simulink model "LM_TOS_0115"  (R2018b)
settings: Solver=FixedStepDiscrete  StartTime=0.0  StopTime=inf  FixedStep=0.005  RelTol=1e-3
PostLoadFcn:
  | if any(exist('dsrtsu_mdlpostloadfcn', 'file') ~= 0), dsrtsu_mdlpostloadfcn('Execute', bdroot); end
(part 1 of 4)
settings Model: DSRTSU_INTERNAL_RTI_VER=540  DSRTSU_INTERNAL_RTI_TYPE=rti1401  RTICANMMDATA=struct('GeneralSetupData',struct('modelroot','D:\00_Work\00_ZOP\00_ZOP_Demo_sim\LaneModel_20210114_CYX_Fix_HWA_TAR_OBJ','generalsettings',struct('filesettings',struct('destfolder',struct('Name','RTICANMM_FILES','Check',1),'buildfolder',struct('Name','.','Check',1),'AbsDestfolder',struct('Name','D:\00_Work\00_ZOP\00_ZOP_Demo_sim\LaneModel_20210114_CYX_Fix_HWA_TAR_OBJ\RTICANMM_FILES'),'AbsBuildfolder',struct('Name','D:\00_Work\00_ZOP\00_ZOP_Demo_sim\LaneModel_20210114_CYX_Fix_HWA_TAR_OBJ'))),'options',struct('addpaths',1,'rmpaths',1,'addtrcexclusion',logical(1),'cannavigator',struct('checkmonitoring',0),'show_usrtrc',0,'use_usrtrc',0),'advanced',struct('options',ones(1,100)),'MPSetup',{{}},'RTI',struct('Type','RTI1401','Ver','7.12','Date','02-May-2019'),'modelname','LM_TOS','block','LM_TOS'))  DSRTSU_INTERNAL_RTIFPGA=130  Creator=only  LastModifiedBy=only
settings OptimizationCC: BlockReduction=off  ConditionallyExecuteInputs=off  DefaultUnderspecifiedDataType=single  BufferReuse=off  EnhancedBackFolding=on  ExpressionFolding=off  PassReuseOutputArgsThreshold=0  LocalBlockOutputs=off  OptimizeBlockOrder=speed  DifferentSizesBufferReuse=on
settings DebuggingCC: ParameterTunabilityLossMsg=error
settings HardwareCC: ProdBitPerPointer=32  ProdBitPerSizeT=32  ProdBitPerPtrDiffT=32  ProdLargestAtomicInteger=Integer  ProdEndianess=BigEndian  ProdWordSize=32  ProdHWDeviceType=Custom Processor->Custom  TargetIntDivRoundTo=Zero  TargetEndianess=BigEndian  TargetHWDeviceType=Custom Processor->Custom
settings ModelReferenceCC: ModelReferenceNumInstancesAllowed=Single
settings SFSimCC: MATLABDynamicMemAlloc=off
settings RTWCC: SystemTargetFile=rti1401.tlc  MakeCommand=make_rti  TemplateMakefile=rti1401.tmf  Description=dSPACE DS1401 Hardware Platform  GenerateReport=on  LaunchReport=on
settings CodeAppCC: OperatorAnnotations=on
settings STFCustomTargetCC: ParMdlRefBuildCompliant=on  SystemTargetFile=rti1401.tlc
settings GRTTargetCC: TargetLangStandard=C89/C90 (ANSI)  CompOptLevelCompliant=off  ConcurrentExecutionCompliant=off  CombineOutputUpdateFcns=off  MatFileLogging=off  CPPClassGenCompliant=off  UseToolchainInfoCompliant=off

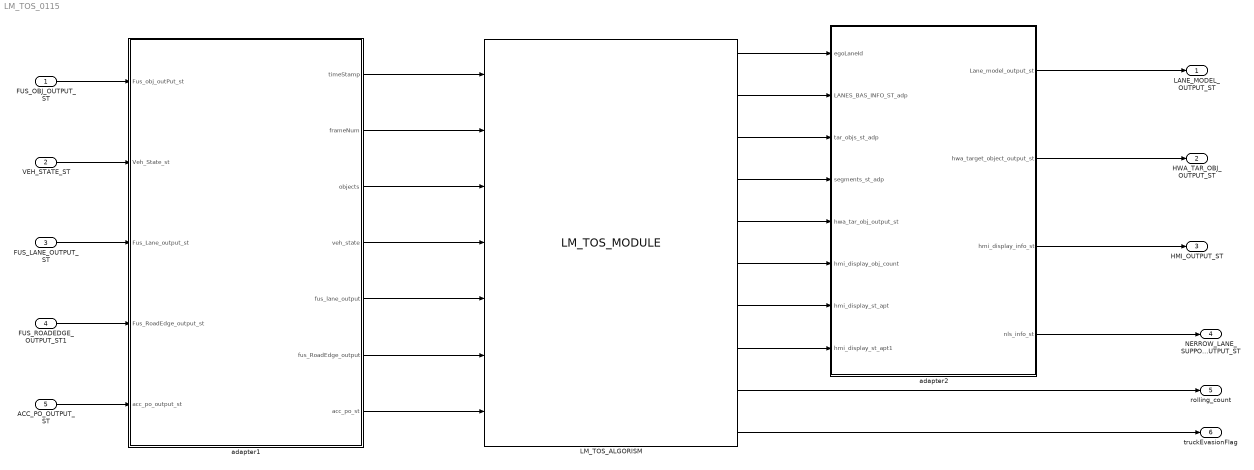
== system LM_TOS_0115 ==
  FUS_OBJ_OUTPUT_ST : Inport  OutDataTypeStr=Bus: FUS_OBJ_OUTPUT_ST
  VEH_STATE_ST : Inport  Port=2  OutDataTypeStr=Bus: VSI_VEHSTATE_ST
  FUS_LANE_OUTPUT_ST : Inport  Port=3  OutDataTypeStr=Bus: FUS_LANE_OUTPUT_ST
  FUS_ROADEDGE_OUTPUT_ST1 : Inport  Port=4  OutDataTypeStr=Bus: FUS_ROAD_EDGE_OUTPUT_ST
  ACC_PO_OUTPUT_ST : Inport  Port=5  OutDataTypeStr=Bus: ATS_PO_ST
  LM_TOS_ALGORISM : S-Function  InitFcn=try, set_param(gcb,'FunctionName','LM_TOS_MODULE'), end  FunctionName=LM_TOS_MODULE  SFunctionModules=LM_TOS_MODULE_wrapper Adapters LMBase LMMathLib LMPp LMTOSRunAlgo LMF TOSBase TOSHWA TOSPp VSL TOSNRA TOSTruckEvasion HMI CoordinationTransformation Parameters VehicleMovement DrivingManeuver LMCommonDefines  SFunctionDeploymentMode=off  EnableBusSupport=off  mask(S-Function Builder){}
      mask help: Simulink:masks:SFunctionBuilder_MD
      mask init:
      | val = [[.9  0.75 0.75 1 1 .9 .9 1]',[1 1 0.75 0.75 .9 .9 1 .9]'];try , sys = get_param(gcb,'SfunBuilderFcnName');if isempty(sys), sys = get_param(gcb,'FunctionName'); end,catch, sys = get_param(gcb,'FunctionName'); end
      settings: CopyFcn=set_param(gcbh,'LinkStatus','none')  PreSaveFcn=try, set_param(gcb,'FunctionName','LM_TOS_MODULE'), end  OpenFcn=sfunctionwizard(gcbh)
      mask Display: plot(val(:,1),val(:,2)),disp(sys), port_label('input',1,'timeStamp_In'), port_label('input',2,'frameNum_In'), port_label('input',3,'objects_In'), port_label('input',4,'vehState_In'), port_label('input',5,'fus_Lane_In'), port_label('input',6,'fus_roadEdge_In'), port_label('input',7,'acc_to_In'), port_label('output',1,'egoLaneId_output'), port_label('output',2,'lanes_bas_info_st_output'), port_label('output',3,'tar_obj_st_output'), port_label('output',4,'segments_st_output'), port_label('output',5,'hwa_tar_obj_st_output'), port_label('output',6,'hmi_obj_count_output'), port_label('output',7,'hmi_info_st_output'), port_label('output',8,'nls_info_st_output'), port_label('output',9,'rolling_count_output'), port_label('output',10,'te_Flag_output')
  adapter1 : Subsystem
  adapter2 : Subsystem
  LANE_MODEL_OUTPUT_ST : Outport  OutDataTypeStr=Bus: LANEMODEL_OUTPUT_ST
  HWA_TAR_OBJ_OUTPUT_ST : Outport  Port=2  OutDataTypeStr=Bus: HWA_TARGETOBJECT_OUTPUT_ST
  HMI_OUTPUT_ST : Outport  Port=3  OutDataTypeStr=Bus: HMI_OUTPUT_ST
  NERROW_LANE_SUPPORT_OUTPUT_ST : Outport  Port=4  OutDataTypeStr=Bus: NARROW_LANE_SUPPORT_OUTPUT_ST
  rolling_count : Outport  Port=5  OutDataTypeStr=uint16
  truckEvasionFlag : Outport  Port=6  OutDataTypeStr=uint8
  wires:
  LM_TOS_ALGORISM/4 -> adapter2/4(segments_st_adp)
  adapter2/2(hwa_target_object_output_st) -> HWA_TAR_OBJ_OUTPUT_ST/1
  adapter1/5(fus_lane_output) -> LM_TOS_ALGORISM/5
  adapter1/2(frameNum) -> LM_TOS_ALGORISM/2
  adapter1/3(objects) -> LM_TOS_ALGORISM/3
  FUS_OBJ_OUTPUT_ST/1 -> adapter1/1(Fus_obj_outPut_st)
  adapter1/1(timeStamp) -> LM_TOS_ALGORISM/1
  adapter1/4(veh_state) -> LM_TOS_ALGORISM/4
  adapter2/1(Lane_model_output_st) -> LANE_MODEL_OUTPUT_ST/1
  LM_TOS_ALGORISM/2 -> adapter2/2(LANES_BAS_INFO_ST_adp)
  FUS_LANE_OUTPUT_ST/1 -> adapter1/3(Fus_Lane_output_st)
  adapter1/7(acc_po_st) -> LM_TOS_ALGORISM/7
  adapter2/4(nls_info_st) -> NERROW_LANE_SUPPORT_OUTPUT_ST/1
  LM_TOS_ALGORISM/10 -> truckEvasionFlag/1
  LM_TOS_ALGORISM/9 -> rolling_count/1
  LM_TOS_ALGORISM/7 -> adapter2/7(hmi_display_st_apt)
  LM_TOS_ALGORISM/6 -> adapter2/6(hmi_display_obj_count)
  LM_TOS_ALGORISM/1 -> adapter2/1(egoLaneId)
  ACC_PO_OUTPUT_ST/1 -> adapter1/5(acc_po_output_st)
  LM_TOS_ALGORISM/3 -> adapter2/3(tar_objs_st_adp)
  adapter2/3(hmi_display_info_st) -> HMI_OUTPUT_ST/1
  LM_TOS_ALGORISM/8 -> adapter2/8(hmi_display_st_apt1)
  adapter1/6(fus_RoadEdge_output) -> LM_TOS_ALGORISM/6
  VEH_STATE_ST/1 -> adapter1/2(Veh_State_st)
  FUS_ROADEDGE_OUTPUT_ST1/1 -> adapter1/4(Fus_RoadEdge_output_st)
  LM_TOS_ALGORISM/5 -> adapter2/5(hwa_tar_obj_output_st)

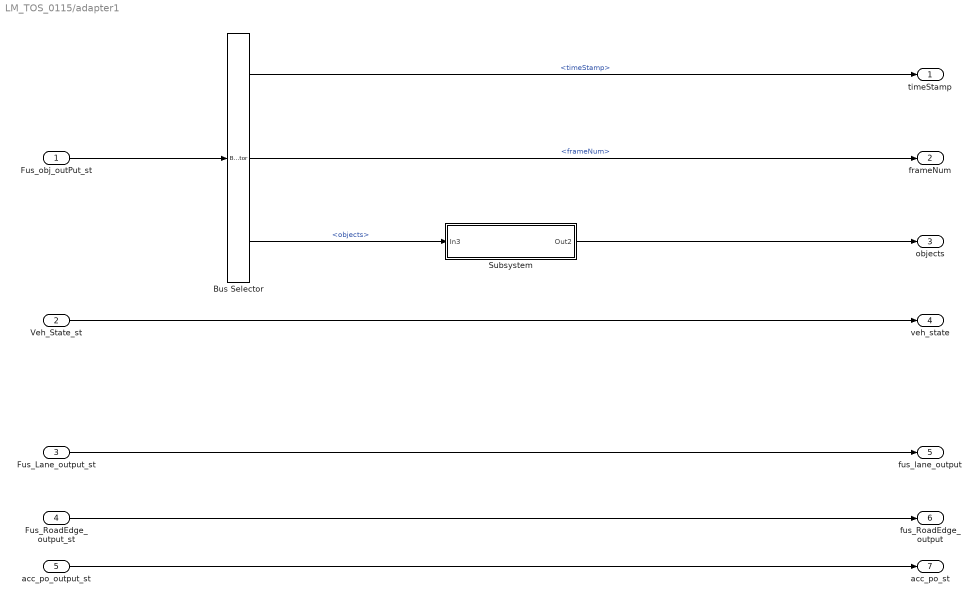
== system LM_TOS_0115/adapter1 ==
  Fus_obj_outPut_st : Inport  OutDataTypeStr=Bus: FUS_OBJ_OUTPUT_ST
  Veh_State_st : Inport  Port=2  OutDataTypeStr=Bus: VSI_VEHSTATE_ST
  Fus_Lane_output_st : Inport  Port=3  OutDataTypeStr=Bus: FUS_LANE_OUTPUT_ST
  Fus_RoadEdge_output_st : Inport  Port=4  OutDataTypeStr=Bus: FUS_ROAD_EDGE_OUTPUT_ST
  acc_po_output_st : Inport  Port=5  OutDataTypeStr=Bus: ATS_PO_ST
  Bus Selector : BusSelector  OutputSignals=timeStamp,frameNum,objects
  Subsystem : Subsystem
  timeStamp : Outport
  frameNum : Outport  Port=2
  objects : Outport  Port=3
  veh_state : Outport  Port=4
  fus_lane_output : Outport  Port=5
  fus_RoadEdge_output : Outport  Port=6  OutDataTypeStr=Bus: FUS_ROAD_EDGE_OUTPUT_ST
  acc_po_st : Outport  Port=7  OutDataTypeStr=Bus: ATS_PO_ST
  wires:
  Fus_obj_outPut_st/1 -> Bus Selector/1
  Bus Selector/3 -> Subsystem/1(In3)  "<objects>"
  Bus Selector/1 -> timeStamp/1  "<timeStamp>"
  Bus Selector/2 -> frameNum/1  "<frameNum>"
  Subsystem/1(Out2) -> objects/1
  Veh_State_st/1 -> veh_state/1
  Fus_Lane_output_st/1 -> fus_lane_output/1
  Fus_RoadEdge_output_st/1 -> fus_RoadEdge_output/1
  acc_po_output_st/1 -> acc_po_st/1

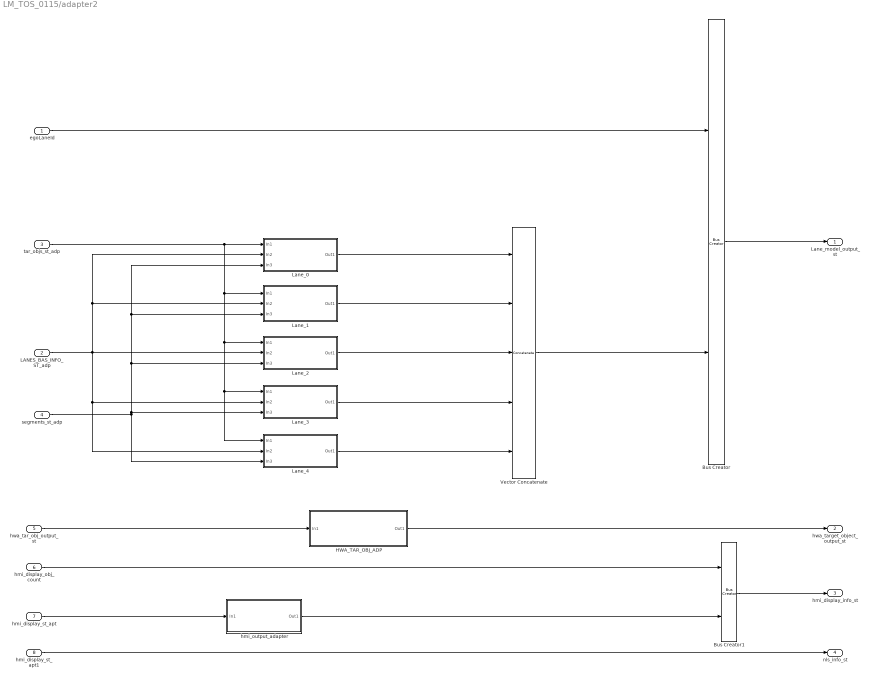
== system LM_TOS_0115/adapter2 ==
  egoLaneId : Inport  OutDataTypeStr=uint8
  LANES_BAS_INFO_ST_adp : Inport  Port=2  OutDataTypeStr=Bus: LANES_BAS_INFO_ST_adt
  tar_objs_st_adp : Inport  Port=3  OutDataTypeStr=Bus: TARGETOBJECTS_ST_adp
  segments_st_adp : Inport  Port=4  OutDataTypeStr=Bus: SEGMENTS_ST_adp
  hwa_tar_obj_output_st : Inport  Port=5  OutDataTypeStr=Bus: HWA_TARGETOBJECT_OUTPUT_ADAPTER_ST
  hmi_display_obj_count : Inport  Port=6  OutDataTypeStr=uint8
  hmi_display_st_apt : Inport  Port=7  OutDataTypeStr=Bus: HMI_OUTPUT_ST_APT
  hmi_display_st_apt1 : Inport  Port=8  OutDataTypeStr=Bus: NARROW_LANE_SUPPORT_OUTPUT_ST
  Bus Creator : BusCreator  Inputs=2
  Bus Creator1 : BusCreator  Inputs=2
  HWA_TAR_OBJ_ADP : Subsystem
  Lane_0 : Subsystem
  Lane_1 : Subsystem
  Lane_2 : Subsystem
  Lane_3 : Subsystem
  Lane_4 : Subsystem
  Vector Concatenate : Concatenate  NumInputs=5
  hmi_output_adapter : Subsystem
  Lane_model_output_st : Outport  OutDataTypeStr=Bus: LANEMODEL_OUTPUT_ST
  hwa_target_object_output_st : Outport  Port=2  OutDataTypeStr=Bus: HWA_TARGETOBJECT_OUTPUT_ST
  hmi_display_info_st : Outport  Port=3  OutDataTypeStr=Bus: HMI_OUTPUT_ST
  nls_info_st : Outport  Port=4  OutDataTypeStr=Bus: NARROW_LANE_SUPPORT_OUTPUT_ST
  wires:
  hwa_tar_obj_output_st/1 -> HWA_TAR_OBJ_ADP/1(In1)
  egoLaneId/1 -> Bus Creator/1
  tar_objs_st_adp/1 -> Lane_0/1(In1), Lane_2/1(In1), Lane_4/1(In1), Lane_3/1(In1), Lane_1/1(In1)
  LANES_BAS_INFO_ST_adp/1 -> Lane_4/2(In2), Lane_3/2(In2), Lane_2/2(In2), Lane_1/2(In2), Lane_0/2(In2)
  segments_st_adp/1 -> Lane_3/3(In3), Lane_2/3(In3), Lane_1/3(In3), Lane_0/3(In3), Lane_4/3(In3)
  Lane_1/1(Out1) -> Vector Concatenate/2
  Lane_2/1(Out1) -> Vector Concatenate/3
  Lane_0/1(Out1) -> Vector Concatenate/1
  Lane_3/1(Out1) -> Vector Concatenate/4
  Lane_4/1(Out1) -> Vector Concatenate/5
  Vector Concatenate/1 -> Bus Creator/2
  Bus Creator/1 -> Lane_model_output_st/1
  hmi_display_st_apt/1 -> hmi_output_adapter/1(In1)
  Bus Creator1/1 -> hmi_display_info_st/1
  hmi_display_obj_count/1 -> Bus Creator1/1
  hmi_output_adapter/1(Out1) -> Bus Creator1/2
  hmi_display_st_apt1/1 -> nls_info_st/1
  HWA_TAR_OBJ_ADP/1(Out1) -> hwa_target_object_output_st/1

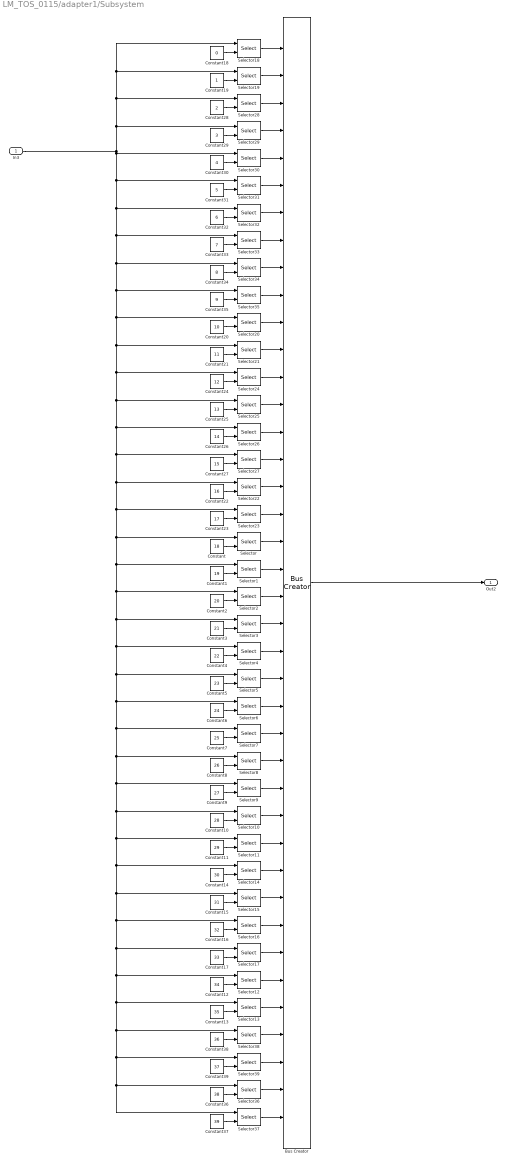
== system LM_TOS_0115/adapter1/Subsystem ==
  In3 : Inport
  Bus Creator : BusCreator  Inputs=40
  Constant : Constant  Value=18
  Constant1 : Constant  Value=19
  Constant10 : Constant  Value=28
  Constant11 : Constant  Value=29
  Constant12 : Constant  Value=34
  Constant13 : Constant  Value=35
  Constant14 : Constant  Value=30
  Constant15 : Constant  Value=31
  Constant16 : Constant  Value=32
  Constant17 : Constant  Value=33
  Constant18 : Constant  Value=0
  Constant19 : Constant
  Constant2 : Constant  Value=20
  Constant20 : Constant  Value=10
  Constant21 : Constant  Value=11
  Constant22 : Constant  Value=16
  Constant23 : Constant  Value=17
  Constant24 : Constant  Value=12
  Constant25 : Constant  Value=13
  Constant26 : Constant  Value=14
  Constant27 : Constant  Value=15
  Constant28 : Constant  Value=2
  Constant29 : Constant  Value=3
  Constant3 : Constant  Value=21
  Constant30 : Constant  Value=4
  Constant31 : Constant  Value=5
  Constant32 : Constant  Value=6
  Constant33 : Constant  Value=7
  Constant34 : Constant  Value=8
  Constant35 : Constant  Value=9
  Constant36 : Constant  Value=38
  Constant37 : Constant  Value=39
  Constant38 : Constant  Value=36
  Constant39 : Constant  Value=37
  Constant4 : Constant  Value=22
  Constant5 : Constant  Value=23
  Constant6 : Constant  Value=24
  Constant7 : Constant  Value=25
  Constant8 : Constant  Value=26
  Constant9 : Constant  Value=27
  Selector{,1..39} (40 alike) : Selector  IndexMode=Zero-based  InputPortWidth=40  IndexOptions=Index vector (port)  Indices=[1 3]  OutputSizes=1
  Out2 : Outport
  wires:
  Constant/1 -> Selector/2
  Constant1/1 -> Selector1/2
  Constant2/1 -> Selector2/2
  Constant5/1 -> Selector5/2
  Constant4/1 -> Selector4/2
  Constant3/1 -> Selector3/2
  Constant9/1 -> Selector9/2
  Constant10/1 -> Selector10/2
  Constant11/1 -> Selector11/2
  Constant8/1 -> Selector8/2
  Constant7/1 -> Selector7/2
  Constant6/1 -> Selector6/2
  Constant14/1 -> Selector14/2
  Constant15/1 -> Selector15/2
  Constant16/1 -> Selector16/2
  Constant13/1 -> Selector13/2
  Constant12/1 -> Selector12/2
  Constant17/1 -> Selector17/2
  Constant27/1 -> Selector27/2
  Constant22/1 -> Selector22/2
  Constant23/1 -> Selector23/2
  Constant26/1 -> Selector26/2
  Constant25/1 -> Selector25/2
  Constant24/1 -> Selector24/2
  Constant32/1 -> Selector32/2
  Constant33/1 -> Selector33/2
  Constant34/1 -> Selector34/2
  Constant21/1 -> Selector21/2
  Constant20/1 -> Selector20/2
  Constant35/1 -> Selector35/2
  Constant29/1 -> Selector29/2
  Constant30/1 -> Selector30/2
  Constant31/1 -> Selector31/2
  Constant28/1 -> Selector28/2
  Constant19/1 -> Selector19/2
  Constant18/1 -> Selector18/2
  Constant39/1 -> Selector39/2
  Constant36/1 -> Selector36/2
  Constant37/1 -> Selector37/2
  Constant38/1 -> Selector38/2
  In3/1 -> Selector30/1, Selector31/1, Selector32/1, Selector33/1, Selector34/1, Selector35/1, Selector20/1, Selector21/1, Selector24/1, Selector25/1, Selector26/1, Selector27/1, Selector22/1, Selector23/1, Selector/1, Selector1/1, Selector2/1, Selector3/1, Selector4/1, Selector5/1, Selector6/1, Selector7/1, Selector8/1, Selector10/1, Selector11/1, Selector14/1, Selector15/1, Selector16/1, Selector17/1, Selector12/1, Selector13/1, Selector38/1, Selector39/1, Selector36/1, Selector37/1, Selector9/1, Selector19/1, Selector18/1, Selector28/1, Selector29/1
  Bus Creator/1 -> Out2/1
  Selector18/1 -> Bus Creator/1
  Selector19/1 -> Bus Creator/2
  Selector28/1 -> Bus Creator/3
  Selector29/1 -> Bus Creator/4
  Selector30/1 -> Bus Creator/5
  Selector31/1 -> Bus Creator/6
  Selector32/1 -> Bus Creator/7
  Selector33/1 -> Bus Creator/8
  Selector34/1 -> Bus Creator/9
  Selector35/1 -> Bus Creator/10
  Selector20/1 -> Bus Creator/11
  Selector21/1 -> Bus Creator/12
  Selector24/1 -> Bus Creator/13
  Selector25/1 -> Bus Creator/14
  Selector26/1 -> Bus Creator/15
  Selector27/1 -> Bus Creator/16
  Selector22/1 -> Bus Creator/17
  Selector23/1 -> Bus Creator/18
  Selector/1 -> Bus Creator/19
  Selector1/1 -> Bus Creator/20
  Selector2/1 -> Bus Creator/21
  Selector3/1 -> Bus Creator/22
  Selector4/1 -> Bus Creator/23
  Selector5/1 -> Bus Creator/24
  Selector6/1 -> Bus Creator/25
  Selector7/1 -> Bus Creator/26
  Selector8/1 -> Bus Creator/27
  Selector9/1 -> Bus Creator/28
  Selector10/1 -> Bus Creator/29
  Selector11/1 -> Bus Creator/30
  Selector14/1 -> Bus Creator/31
  Selector15/1 -> Bus Creator/32
  Selector16/1 -> Bus Creator/33
  Selector17/1 -> Bus Creator/34
  Selector12/1 -> Bus Creator/35
  Selector13/1 -> Bus Creator/36
  Selector38/1 -> Bus Creator/37
  Selector39/1 -> Bus Creator/38
  Selector36/1 -> Bus Creator/39
  Selector37/1 -> Bus Creator/40

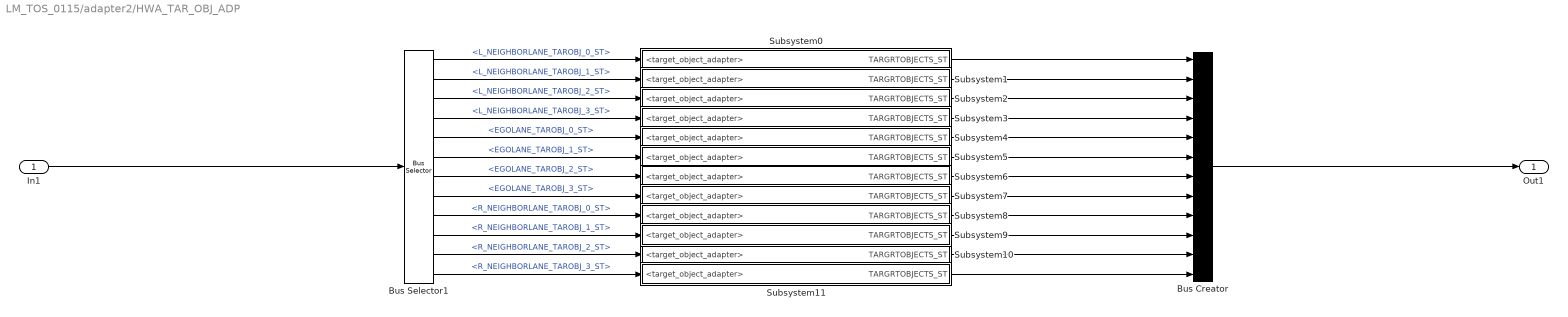
== system LM_TOS_0115/adapter2/HWA_TAR_OBJ_ADP ==
  In1 : Inport
  Bus Creator : BusCreator  Inputs=12  OutDataTypeStr=Bus: HWA_TARGETOBJECT_OUTPUT_ST  NonVirtualBus=on
  Bus Selector1 : BusSelector  OutputSignals=L_NEIGHBORLANE_TAROBJ_0_ST,L_NEIGHBORLANE_TAROBJ_1_ST,L_NEIGHBORLANE_TAROBJ_2_ST,L_NEIGHBORLANE_TAROBJ_3_ST,EGOLANE_TAROBJ_0_ST,EGOLANE_TAROBJ_1_ST,EGOLANE_TAROBJ_2_ST,EGOLANE_TAROBJ_3_ST,R_NEIGHBORLANE_TAROBJ_0_ST,R_NEIGHBORLANE_TAROBJ_1_ST,R_NEIGHBORLANE_TAROBJ_2_ST,R_NEIGHBORLANE_TAROBJ_3_ST
  Subsystem0 : Subsystem
  Subsystem1 : Subsystem
  Subsystem10 : Subsystem
  Subsystem11 : Subsystem
  Subsystem2 : Subsystem
  Subsystem3 : Subsystem
  Subsystem4 : Subsystem
  Subsystem5 : Subsystem
  Subsystem6 : Subsystem
  Subsystem7 : Subsystem
  Subsystem8 : Subsystem
  Subsystem9 : Subsystem
  Out1 : Outport  OutDataTypeStr=Bus: HWA_TARGETOBJECT_OUTPUT_ST
  wires:
  In1/1 -> Bus Selector1/1
  Bus Selector1/1 -> Subsystem0/1(<target_object_adapter>)  "<L_NEIGHBORLANE_TAROBJ_0_ST>"
  Bus Selector1/2 -> Subsystem1/1(<target_object_adapter>)  "<L_NEIGHBORLANE_TAROBJ_1_ST>"
  Bus Selector1/3 -> Subsystem2/1(<target_object_adapter>)  "<L_NEIGHBORLANE_TAROBJ_2_ST>"
  Bus Selector1/4 -> Subsystem3/1(<target_object_adapter>)  "<L_NEIGHBORLANE_TAROBJ_3_ST>"
  Bus Selector1/5 -> Subsystem4/1(<target_object_adapter>)  "<EGOLANE_TAROBJ_0_ST>"
  Bus Selector1/6 -> Subsystem5/1(<target_object_adapter>)  "<EGOLANE_TAROBJ_1_ST>"
  Bus Selector1/7 -> Subsystem6/1(<target_object_adapter>)  "<EGOLANE_TAROBJ_2_ST>"
  Bus Selector1/8 -> Subsystem7/1(<target_object_adapter>)  "<EGOLANE_TAROBJ_3_ST>"
  Bus Selector1/9 -> Subsystem8/1(<target_object_adapter>)  "<R_NEIGHBORLANE_TAROBJ_0_ST>"
  Bus Selector1/10 -> Subsystem9/1(<target_object_adapter>)  "<R_NEIGHBORLANE_TAROBJ_1_ST>"
  Bus Selector1/11 -> Subsystem10/1(<target_object_adapter>)  "<R_NEIGHBORLANE_TAROBJ_2_ST>"
  Bus Selector1/12 -> Subsystem11/1(<target_object_adapter>)  "<R_NEIGHBORLANE_TAROBJ_3_ST>"
  Subsystem0/1(TARGRTOBJECTS_ST) -> Bus Creator/1
  Subsystem1/1(TARGRTOBJECTS_ST) -> Bus Creator/2
  Subsystem2/1(TARGRTOBJECTS_ST) -> Bus Creator/3
  Subsystem3/1(TARGRTOBJECTS_ST) -> Bus Creator/4
  Subsystem4/1(TARGRTOBJECTS_ST) -> Bus Creator/5
  Subsystem5/1(TARGRTOBJECTS_ST) -> Bus Creator/6
  Subsystem6/1(TARGRTOBJECTS_ST) -> Bus Creator/7
  Subsystem7/1(TARGRTOBJECTS_ST) -> Bus Creator/8
  Subsystem8/1(TARGRTOBJECTS_ST) -> Bus Creator/9
  Subsystem9/1(TARGRTOBJECTS_ST) -> Bus Creator/10
  Subsystem10/1(TARGRTOBJECTS_ST) -> Bus Creator/11
  Subsystem11/1(TARGRTOBJECTS_ST) -> Bus Creator/12
  Bus Creator/1 -> Out1/1

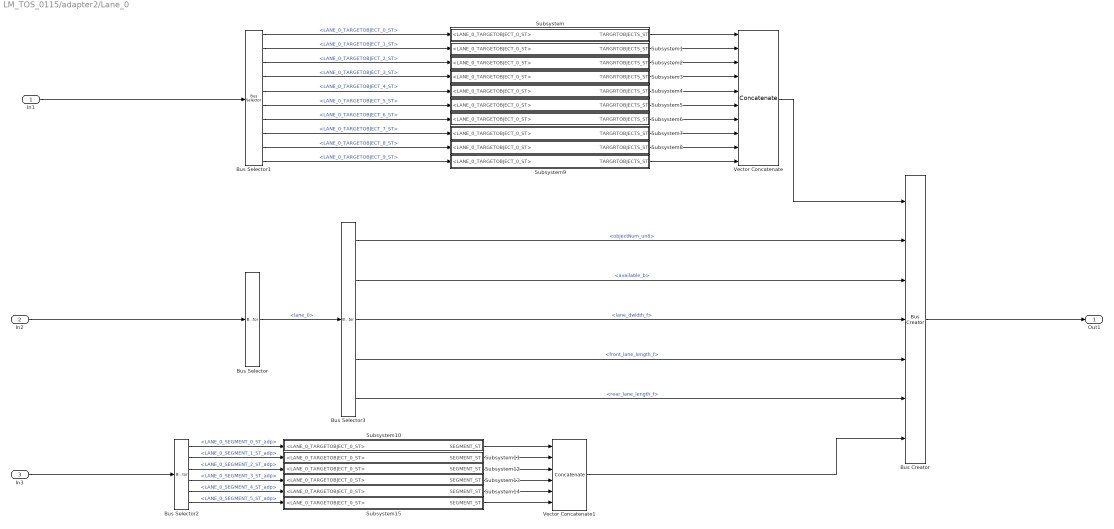
== system LM_TOS_0115/adapter2/Lane_0 ==
  In1 : Inport
  In2 : Inport  Port=2
  In3 : Inport  Port=3
  Bus Creator : BusCreator  Inputs=7  OutDataTypeStr=Bus: LM_LANE_ST  NonVirtualBus=on
  Bus Selector : BusSelector  OutputSignals=lane_0
  Bus Selector1 : BusSelector  OutputSignals=LANE_0_TARGETOBJECT_0_ST,LANE_0_TARGETOBJECT_1_ST,LANE_0_TARGETOBJECT_2_ST,LANE_0_TARGETOBJECT_3_ST,LANE_0_TARGETOBJECT_4_ST,LANE_0_TARGETOBJECT_5_ST,LANE_0_TARGETOBJECT_6_ST,LANE_0_TARGETOBJECT_7_ST,LANE_0_TARGETOBJECT_8_ST,LANE_0_TARGETOBJECT_9_ST
  Bus Selector2 : BusSelector  OutputSignals=LANE_0_SEGMENT_0_ST_adp,LANE_0_SEGMENT_1_ST_adp,LANE_0_SEGMENT_2_ST_adp,LANE_0_SEGMENT_3_ST_adp,LANE_0_SEGMENT_4_ST_adp,LANE_0_SEGMENT_5_ST_adp
  Bus Selector3 : BusSelector  OutputSignals=objectNum_un8,available_b,lane_dwidth_f,front_lane_length_f,rear_lane_length_f
  Subsystem : Subsystem
  Subsystem1 : Subsystem
  Subsystem10 : Subsystem
  Subsystem11 : Subsystem
  Subsystem12 : Subsystem
  Subsystem13 : Subsystem
  Subsystem14 : Subsystem
  Subsystem15 : Subsystem
  Subsystem2 : Subsystem
  Subsystem3 : Subsystem
  Subsystem4 : Subsystem
  Subsystem5 : Subsystem
  Subsystem6 : Subsystem
  Subsystem7 : Subsystem
  Subsystem8 : Subsystem
  Subsystem9 : Subsystem
  Vector Concatenate : Concatenate  NumInputs=10
  Vector Concatenate1 : Concatenate  NumInputs=6
  Out1 : Outport  OutDataTypeStr=Bus: LM_LANE_ST
  wires:
  Bus Selector2/4 -> Subsystem13/1(<LANE_0_TARGETOBJECT_0_ST>)  "<LANE_0_SEGMENT_3_ST_adp>"
  Subsystem9/1(TARGRTOBJECTS_ST) -> Vector Concatenate/10
  Subsystem7/1(TARGRTOBJECTS_ST) -> Vector Concatenate/8
  Bus Selector1/8 -> Subsystem7/1(<LANE_0_TARGETOBJECT_0_ST>)  "<LANE_0_TARGETOBJECT_7_ST>"
  Subsystem15/1(SEGMENT_ST) -> Vector Concatenate1/6
  Subsystem2/1(TARGRTOBJECTS_ST) -> Vector Concatenate/3
  Subsystem10/1(SEGMENT_ST) -> Vector Concatenate1/1
  Subsystem11/1(SEGMENT_ST) -> Vector Concatenate1/2
  Subsystem8/1(TARGRTOBJECTS_ST) -> Vector Concatenate/9
  Subsystem6/1(TARGRTOBJECTS_ST) -> Vector Concatenate/7
  Bus Selector3/3 -> Bus Creator/4  "<lane_dwidth_f>"
  Subsystem12/1(SEGMENT_ST) -> Vector Concatenate1/3
  Subsystem5/1(TARGRTOBJECTS_ST) -> Vector Concatenate/6
  Subsystem13/1(SEGMENT_ST) -> Vector Concatenate1/4
  Subsystem14/1(SEGMENT_ST) -> Vector Concatenate1/5
  Subsystem4/1(TARGRTOBJECTS_ST) -> Vector Concatenate/5
  Bus Creator/1 -> Out1/1
  Bus Selector1/10 -> Subsystem9/1(<LANE_0_TARGETOBJECT_0_ST>)  "<LANE_0_TARGETOBJECT_9_ST>"
  Subsystem1/1(TARGRTOBJECTS_ST) -> Vector Concatenate/2
  Bus Selector1/2 -> Subsystem1/1(<LANE_0_TARGETOBJECT_0_ST>)  "<LANE_0_TARGETOBJECT_1_ST>"
  Bus Selector2/3 -> Subsystem12/1(<LANE_0_TARGETOBJECT_0_ST>)  "<LANE_0_SEGMENT_2_ST_adp>"
  Bus Selector3/2 -> Bus Creator/3  "<available_b>"
  Bus Selector/1 -> Bus Selector3/1  "<lane_0>"
  Bus Selector1/9 -> Subsystem8/1(<LANE_0_TARGETOBJECT_0_ST>)  "<LANE_0_TARGETOBJECT_8_ST>"
  Bus Selector1/7 -> Subsystem6/1(<LANE_0_TARGETOBJECT_0_ST>)  "<LANE_0_TARGETOBJECT_6_ST>"
  Bus Selector1/3 -> Subsystem2/1(<LANE_0_TARGETOBJECT_0_ST>)  "<LANE_0_TARGETOBJECT_2_ST>"
  Bus Selector2/6 -> Subsystem15/1(<LANE_0_TARGETOBJECT_0_ST>)  "<LANE_0_SEGMENT_5_ST_adp>"
  Bus Selector1/5 -> Subsystem4/1(<LANE_0_TARGETOBJECT_0_ST>)  "<LANE_0_TARGETOBJECT_4_ST>"
  Bus Selector3/5 -> Bus Creator/6  "<rear_lane_length_f>"
  Bus Selector2/5 -> Subsystem14/1(<LANE_0_TARGETOBJECT_0_ST>)  "<LANE_0_SEGMENT_4_ST_adp>"
  Bus Selector2/2 -> Subsystem11/1(<LANE_0_TARGETOBJECT_0_ST>)  "<LANE_0_SEGMENT_1_ST_adp>"
  Bus Selector2/1 -> Subsystem10/1(<LANE_0_TARGETOBJECT_0_ST>)  "<LANE_0_SEGMENT_0_ST_adp>"
  In1/1 -> Bus Selector1/1
  In3/1 -> Bus Selector2/1
  Bus Selector1/6 -> Subsystem5/1(<LANE_0_TARGETOBJECT_0_ST>)  "<LANE_0_TARGETOBJECT_5_ST>"
  Bus Selector1/1 -> Subsystem/1(<LANE_0_TARGETOBJECT_0_ST>)  "<LANE_0_TARGETOBJECT_0_ST>"
  Bus Selector1/4 -> Subsystem3/1(<LANE_0_TARGETOBJECT_0_ST>)  "<LANE_0_TARGETOBJECT_3_ST>"
  Bus Selector3/1 -> Bus Creator/2  "<objectNum_un8>"
  Bus Selector3/4 -> Bus Creator/5  "<front_lane_length_f>"
  Subsystem/1(TARGRTOBJECTS_ST) -> Vector Concatenate/1
  Vector Concatenate/1 -> Bus Creator/1
  Subsystem3/1(TARGRTOBJECTS_ST) -> Vector Concatenate/4
  Vector Concatenate1/1 -> Bus Creator/7
  In2/1 -> Bus Selector/1

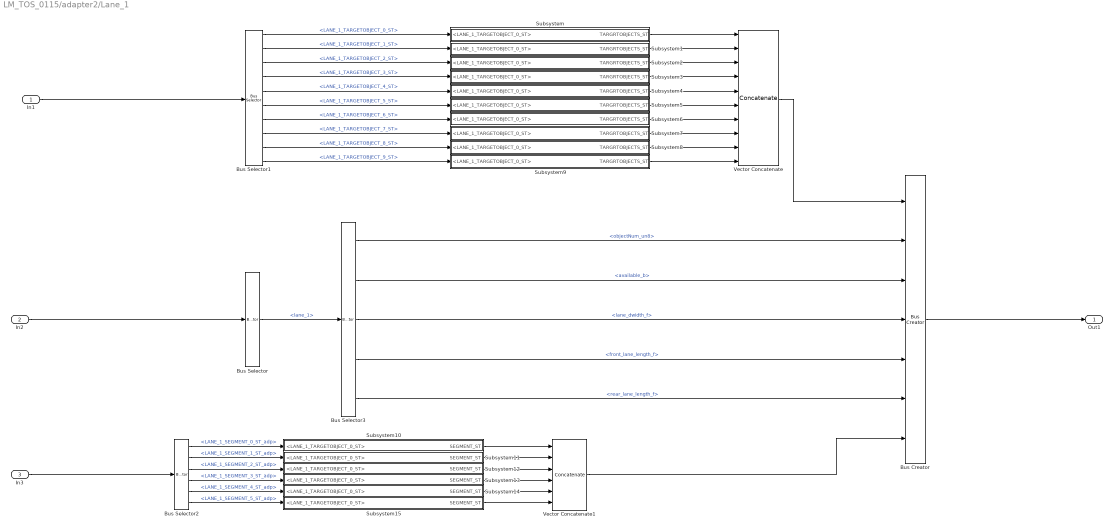
== system LM_TOS_0115/adapter2/Lane_1 ==
  In1 : Inport
  In2 : Inport  Port=2
  In3 : Inport  Port=3
  Bus Creator : BusCreator  Inputs=7  OutDataTypeStr=Bus: LM_LANE_ST  NonVirtualBus=on
  Bus Selector : BusSelector  OutputSignals=lane_1
  Bus Selector1 : BusSelector  OutputSignals=LANE_1_TARGETOBJECT_0_ST,LANE_1_TARGETOBJECT_1_ST,LANE_1_TARGETOBJECT_2_ST,LANE_1_TARGETOBJECT_3_ST,LANE_1_TARGETOBJECT_4_ST,LANE_1_TARGETOBJECT_5_ST,LANE_1_TARGETOBJECT_6_ST,LANE_1_TARGETOBJECT_7_ST,LANE_1_TARGETOBJECT_8_ST,LANE_1_TARGETOBJECT_9_ST
  Bus Selector2 : BusSelector  OutputSignals=LANE_1_SEGMENT_0_ST_adp,LANE_1_SEGMENT_1_ST_adp,LANE_1_SEGMENT_2_ST_adp,LANE_1_SEGMENT_3_ST_adp,LANE_1_SEGMENT_4_ST_adp,LANE_1_SEGMENT_5_ST_adp
  Bus Selector3 : BusSelector  OutputSignals=objectNum_un8,available_b,lane_dwidth_f,front_lane_length_f,rear_lane_length_f
  Subsystem : Subsystem
  Subsystem1 : Subsystem
  Subsystem10 : Subsystem
  Subsystem11 : Subsystem
  Subsystem12 : Subsystem
  Subsystem13 : Subsystem
  Subsystem14 : Subsystem
  Subsystem15 : Subsystem
  Subsystem2 : Subsystem
  Subsystem3 : Subsystem
  Subsystem4 : Subsystem
  Subsystem5 : Subsystem
  Subsystem6 : Subsystem
  Subsystem7 : Subsystem
  Subsystem8 : Subsystem
  Subsystem9 : Subsystem
  Vector Concatenate : Concatenate  NumInputs=10
  Vector Concatenate1 : Concatenate  NumInputs=6
  Out1 : Outport  OutDataTypeStr=Bus: LM_LANE_ST
  wires:
  In2/1 -> Bus Selector/1
  Vector Concatenate1/1 -> Bus Creator/7
  Subsystem3/1(TARGRTOBJECTS_ST) -> Vector Concatenate/4
  Vector Concatenate/1 -> Bus Creator/1
  Subsystem/1(TARGRTOBJECTS_ST) -> Vector Concatenate/1
  Bus Selector3/4 -> Bus Creator/5  "<front_lane_length_f>"
  Bus Selector3/1 -> Bus Creator/2  "<objectNum_un8>"
  Bus Selector1/4 -> Subsystem3/1(<LANE_1_TARGETOBJECT_0_ST>)  "<LANE_1_TARGETOBJECT_3_ST>"
  Bus Selector1/1 -> Subsystem/1(<LANE_1_TARGETOBJECT_0_ST>)  "<LANE_1_TARGETOBJECT_0_ST>"
  Bus Selector1/6 -> Subsystem5/1(<LANE_1_TARGETOBJECT_0_ST>)  "<LANE_1_TARGETOBJECT_5_ST>"
  In3/1 -> Bus Selector2/1
  In1/1 -> Bus Selector1/1
  Bus Selector2/1 -> Subsystem10/1(<LANE_1_TARGETOBJECT_0_ST>)  "<LANE_1_SEGMENT_0_ST_adp>"
  Bus Selector2/2 -> Subsystem11/1(<LANE_1_TARGETOBJECT_0_ST>)  "<LANE_1_SEGMENT_1_ST_adp>"
  Bus Selector2/5 -> Subsystem14/1(<LANE_1_TARGETOBJECT_0_ST>)  "<LANE_1_SEGMENT_4_ST_adp>"
  Bus Selector3/5 -> Bus Creator/6  "<rear_lane_length_f>"
  Bus Selector1/5 -> Subsystem4/1(<LANE_1_TARGETOBJECT_0_ST>)  "<LANE_1_TARGETOBJECT_4_ST>"
  Bus Selector2/6 -> Subsystem15/1(<LANE_1_TARGETOBJECT_0_ST>)  "<LANE_1_SEGMENT_5_ST_adp>"
  Bus Selector1/3 -> Subsystem2/1(<LANE_1_TARGETOBJECT_0_ST>)  "<LANE_1_TARGETOBJECT_2_ST>"
  Bus Selector1/7 -> Subsystem6/1(<LANE_1_TARGETOBJECT_0_ST>)  "<LANE_1_TARGETOBJECT_6_ST>"
  Bus Selector1/9 -> Subsystem8/1(<LANE_1_TARGETOBJECT_0_ST>)  "<LANE_1_TARGETOBJECT_8_ST>"
  Bus Selector/1 -> Bus Selector3/1  "<lane_1>"
  Bus Selector3/2 -> Bus Creator/3  "<available_b>"
  Bus Selector2/3 -> Subsystem12/1(<LANE_1_TARGETOBJECT_0_ST>)  "<LANE_1_SEGMENT_2_ST_adp>"
  Bus Selector1/2 -> Subsystem1/1(<LANE_1_TARGETOBJECT_0_ST>)  "<LANE_1_TARGETOBJECT_1_ST>"
  Subsystem1/1(TARGRTOBJECTS_ST) -> Vector Concatenate/2
  Bus Selector1/10 -> Subsystem9/1(<LANE_1_TARGETOBJECT_0_ST>)  "<LANE_1_TARGETOBJECT_9_ST>"
  Bus Creator/1 -> Out1/1
  Subsystem4/1(TARGRTOBJECTS_ST) -> Vector Concatenate/5
  Subsystem14/1(SEGMENT_ST) -> Vector Concatenate1/5
  Subsystem13/1(SEGMENT_ST) -> Vector Concatenate1/4
  Subsystem5/1(TARGRTOBJECTS_ST) -> Vector Concatenate/6
  Subsystem12/1(SEGMENT_ST) -> Vector Concatenate1/3
  Bus Selector3/3 -> Bus Creator/4  "<lane_dwidth_f>"
  Subsystem6/1(TARGRTOBJECTS_ST) -> Vector Concatenate/7
  Subsystem8/1(TARGRTOBJECTS_ST) -> Vector Concatenate/9
  Subsystem11/1(SEGMENT_ST) -> Vector Concatenate1/2
  Subsystem10/1(SEGMENT_ST) -> Vector Concatenate1/1
  Subsystem2/1(TARGRTOBJECTS_ST) -> Vector Concatenate/3
  Subsystem15/1(SEGMENT_ST) -> Vector Concatenate1/6
  Bus Selector1/8 -> Subsystem7/1(<LANE_1_TARGETOBJECT_0_ST>)  "<LANE_1_TARGETOBJECT_7_ST>"
  Subsystem7/1(TARGRTOBJECTS_ST) -> Vector Concatenate/8
  Subsystem9/1(TARGRTOBJECTS_ST) -> Vector Concatenate/10
  Bus Selector2/4 -> Subsystem13/1(<LANE_1_TARGETOBJECT_0_ST>)  "<LANE_1_SEGMENT_3_ST_adp>"

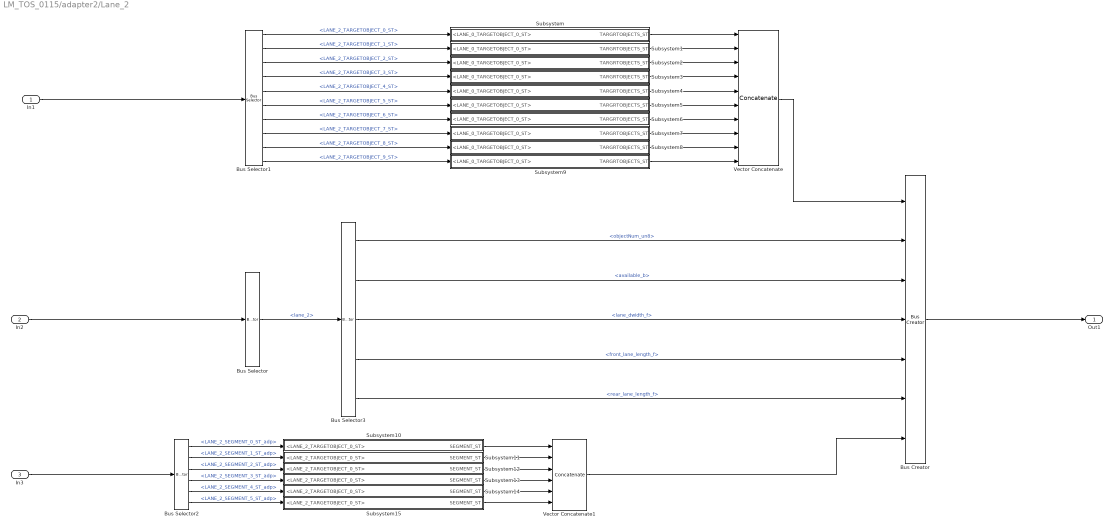
== system LM_TOS_0115/adapter2/Lane_2 ==
  In1 : Inport
  In2 : Inport  Port=2
  In3 : Inport  Port=3
  Bus Creator : BusCreator  Inputs=7  OutDataTypeStr=Bus: LM_LANE_ST  NonVirtualBus=on
  Bus Selector : BusSelector  OutputSignals=lane_2
  Bus Selector1 : BusSelector  OutputSignals=LANE_2_TARGETOBJECT_0_ST,LANE_2_TARGETOBJECT_1_ST,LANE_2_TARGETOBJECT_2_ST,LANE_2_TARGETOBJECT_3_ST,LANE_2_TARGETOBJECT_4_ST,LANE_2_TARGETOBJECT_5_ST,LANE_2_TARGETOBJECT_6_ST,LANE_2_TARGETOBJECT_7_ST,LANE_2_TARGETOBJECT_8_ST,LANE_2_TARGETOBJECT_9_ST
  Bus Selector2 : BusSelector  OutputSignals=LANE_2_SEGMENT_0_ST_adp,LANE_2_SEGMENT_1_ST_adp,LANE_2_SEGMENT_2_ST_adp,LANE_2_SEGMENT_3_ST_adp,LANE_2_SEGMENT_4_ST_adp,LANE_2_SEGMENT_5_ST_adp
  Bus Selector3 : BusSelector  OutputSignals=objectNum_un8,available_b,lane_dwidth_f,front_lane_length_f,rear_lane_length_f
  Subsystem : Subsystem
  Subsystem1 : Subsystem
  Subsystem10 : Subsystem
  Subsystem11 : Subsystem
  Subsystem12 : Subsystem
  Subsystem13 : Subsystem
  Subsystem14 : Subsystem
  Subsystem15 : Subsystem
  Subsystem2 : Subsystem
  Subsystem3 : Subsystem
  Subsystem4 : Subsystem
  Subsystem5 : Subsystem
  Subsystem6 : Subsystem
  Subsystem7 : Subsystem
  Subsystem8 : Subsystem
  Subsystem9 : Subsystem
  Vector Concatenate : Concatenate  NumInputs=10
  Vector Concatenate1 : Concatenate  NumInputs=6
  Out1 : Outport  OutDataTypeStr=Bus: LM_LANE_ST
  wires:
  Bus Selector2/4 -> Subsystem13/1(<LANE_2_TARGETOBJECT_0_ST>)  "<LANE_2_SEGMENT_3_ST_adp>"
  Subsystem9/1(TARGRTOBJECTS_ST) -> Vector Concatenate/10
  Subsystem7/1(TARGRTOBJECTS_ST) -> Vector Concatenate/8
  Bus Selector1/8 -> Subsystem7/1(<LANE_0_TARGETOBJECT_0_ST>)  "<LANE_2_TARGETOBJECT_7_ST>"
  Subsystem15/1(SEGMENT_ST) -> Vector Concatenate1/6
  Subsystem2/1(TARGRTOBJECTS_ST) -> Vector Concatenate/3
  Subsystem10/1(SEGMENT_ST) -> Vector Concatenate1/1
  Subsystem11/1(SEGMENT_ST) -> Vector Concatenate1/2
  Subsystem8/1(TARGRTOBJECTS_ST) -> Vector Concatenate/9
  Subsystem6/1(TARGRTOBJECTS_ST) -> Vector Concatenate/7
  Bus Selector3/3 -> Bus Creator/4  "<lane_dwidth_f>"
  Subsystem12/1(SEGMENT_ST) -> Vector Concatenate1/3
  Subsystem5/1(TARGRTOBJECTS_ST) -> Vector Concatenate/6
  Subsystem13/1(SEGMENT_ST) -> Vector Concatenate1/4
  Subsystem14/1(SEGMENT_ST) -> Vector Concatenate1/5
  Subsystem4/1(TARGRTOBJECTS_ST) -> Vector Concatenate/5
  Bus Creator/1 -> Out1/1
  Bus Selector1/10 -> Subsystem9/1(<LANE_0_TARGETOBJECT_0_ST>)  "<LANE_2_TARGETOBJECT_9_ST>"
  Subsystem1/1(TARGRTOBJECTS_ST) -> Vector Concatenate/2
  Bus Selector1/2 -> Subsystem1/1(<LANE_0_TARGETOBJECT_0_ST>)  "<LANE_2_TARGETOBJECT_1_ST>"
  Bus Selector2/3 -> Subsystem12/1(<LANE_2_TARGETOBJECT_0_ST>)  "<LANE_2_SEGMENT_2_ST_adp>"
  Bus Selector3/2 -> Bus Creator/3  "<available_b>"
  Bus Selector/1 -> Bus Selector3/1  "<lane_2>"
  Bus Selector1/9 -> Subsystem8/1(<LANE_0_TARGETOBJECT_0_ST>)  "<LANE_2_TARGETOBJECT_8_ST>"
  Bus Selector1/7 -> Subsystem6/1(<LANE_0_TARGETOBJECT_0_ST>)  "<LANE_2_TARGETOBJECT_6_ST>"
  Bus Selector1/3 -> Subsystem2/1(<LANE_0_TARGETOBJECT_0_ST>)  "<LANE_2_TARGETOBJECT_2_ST>"
  Bus Selector2/6 -> Subsystem15/1(<LANE_2_TARGETOBJECT_0_ST>)  "<LANE_2_SEGMENT_5_ST_adp>"
  Bus Selector1/5 -> Subsystem4/1(<LANE_0_TARGETOBJECT_0_ST>)  "<LANE_2_TARGETOBJECT_4_ST>"
  Bus Selector3/5 -> Bus Creator/6  "<rear_lane_length_f>"
  Bus Selector2/5 -> Subsystem14/1(<LANE_2_TARGETOBJECT_0_ST>)  "<LANE_2_SEGMENT_4_ST_adp>"
  Bus Selector2/2 -> Subsystem11/1(<LANE_2_TARGETOBJECT_0_ST>)  "<LANE_2_SEGMENT_1_ST_adp>"
  Bus Selector2/1 -> Subsystem10/1(<LANE_2_TARGETOBJECT_0_ST>)  "<LANE_2_SEGMENT_0_ST_adp>"
  In1/1 -> Bus Selector1/1
  In3/1 -> Bus Selector2/1
  Bus Selector1/6 -> Subsystem5/1(<LANE_0_TARGETOBJECT_0_ST>)  "<LANE_2_TARGETOBJECT_5_ST>"
  Bus Selector1/1 -> Subsystem/1(<LANE_0_TARGETOBJECT_0_ST>)  "<LANE_2_TARGETOBJECT_0_ST>"
  Bus Selector1/4 -> Subsystem3/1(<LANE_0_TARGETOBJECT_0_ST>)  "<LANE_2_TARGETOBJECT_3_ST>"
  Bus Selector3/1 -> Bus Creator/2  "<objectNum_un8>"
  Bus Selector3/4 -> Bus Creator/5  "<front_lane_length_f>"
  Subsystem/1(TARGRTOBJECTS_ST) -> Vector Concatenate/1
  Vector Concatenate/1 -> Bus Creator/1
  Subsystem3/1(TARGRTOBJECTS_ST) -> Vector Concatenate/4
  Vector Concatenate1/1 -> Bus Creator/7
  In2/1 -> Bus Selector/1

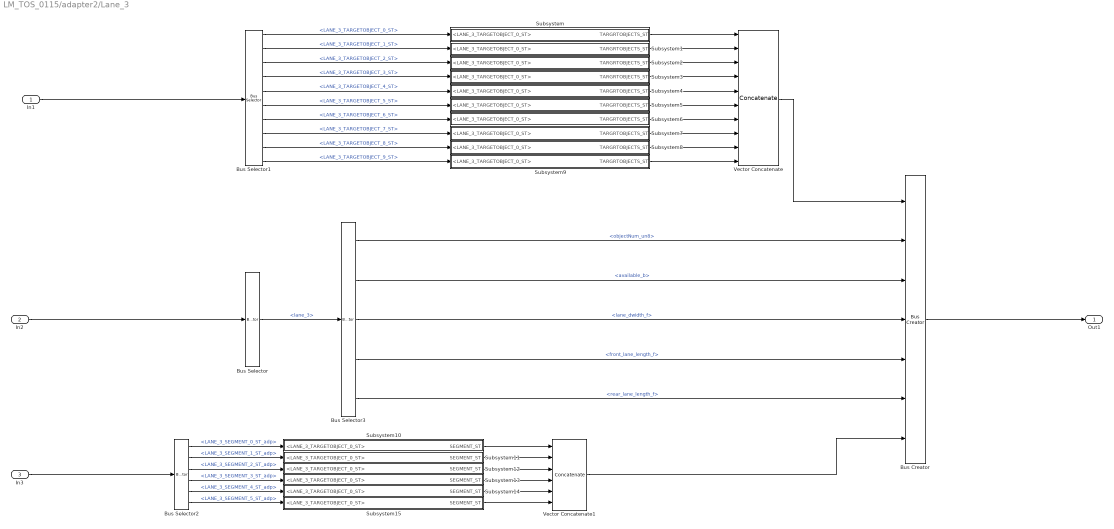
== system LM_TOS_0115/adapter2/Lane_3 ==
  In1 : Inport
  In2 : Inport  Port=2
  In3 : Inport  Port=3
  Bus Creator : BusCreator  Inputs=7  OutDataTypeStr=Bus: LM_LANE_ST  NonVirtualBus=on
  Bus Selector : BusSelector  OutputSignals=lane_3
  Bus Selector1 : BusSelector  OutputSignals=LANE_3_TARGETOBJECT_0_ST,LANE_3_TARGETOBJECT_1_ST,LANE_3_TARGETOBJECT_2_ST,LANE_3_TARGETOBJECT_3_ST,LANE_3_TARGETOBJECT_4_ST,LANE_3_TARGETOBJECT_5_ST,LANE_3_TARGETOBJECT_6_ST,LANE_3_TARGETOBJECT_7_ST,LANE_3_TARGETOBJECT_8_ST,LANE_3_TARGETOBJECT_9_ST
  Bus Selector2 : BusSelector  OutputSignals=LANE_3_SEGMENT_0_ST_adp,LANE_3_SEGMENT_1_ST_adp,LANE_3_SEGMENT_2_ST_adp,LANE_3_SEGMENT_3_ST_adp,LANE_3_SEGMENT_4_ST_adp,LANE_3_SEGMENT_5_ST_adp
  Bus Selector3 : BusSelector  OutputSignals=objectNum_un8,available_b,lane_dwidth_f,front_lane_length_f,rear_lane_length_f
  Subsystem : Subsystem
  Subsystem1 : Subsystem
  Subsystem10 : Subsystem
  Subsystem11 : Subsystem
  Subsystem12 : Subsystem
  Subsystem13 : Subsystem
  Subsystem14 : Subsystem
  Subsystem15 : Subsystem
  Subsystem2 : Subsystem
  Subsystem3 : Subsystem
  Subsystem4 : Subsystem
  Subsystem5 : Subsystem
  Subsystem6 : Subsystem
  Subsystem7 : Subsystem
  Subsystem8 : Subsystem
  Subsystem9 : Subsystem
  Vector Concatenate : Concatenate  NumInputs=10
  Vector Concatenate1 : Concatenate  NumInputs=6
  Out1 : Outport  OutDataTypeStr=Bus: LM_LANE_ST
  wires:
  In2/1 -> Bus Selector/1
  Vector Concatenate1/1 -> Bus Creator/7
  Subsystem3/1(TARGRTOBJECTS_ST) -> Vector Concatenate/4
  Vector Concatenate/1 -> Bus Creator/1
  Subsystem/1(TARGRTOBJECTS_ST) -> Vector Concatenate/1
  Bus Selector3/4 -> Bus Creator/5  "<front_lane_length_f>"
  Bus Selector3/1 -> Bus Creator/2  "<objectNum_un8>"
  Bus Selector1/4 -> Subsystem3/1(<LANE_3_TARGETOBJECT_0_ST>)  "<LANE_3_TARGETOBJECT_3_ST>"
  Bus Selector1/1 -> Subsystem/1(<LANE_3_TARGETOBJECT_0_ST>)  "<LANE_3_TARGETOBJECT_0_ST>"
  Bus Selector1/6 -> Subsystem5/1(<LANE_3_TARGETOBJECT_0_ST>)  "<LANE_3_TARGETOBJECT_5_ST>"
  In3/1 -> Bus Selector2/1
  In1/1 -> Bus Selector1/1
  Bus Selector2/1 -> Subsystem10/1(<LANE_3_TARGETOBJECT_0_ST>)  "<LANE_3_SEGMENT_0_ST_adp>"
  Bus Selector2/2 -> Subsystem11/1(<LANE_3_TARGETOBJECT_0_ST>)  "<LANE_3_SEGMENT_1_ST_adp>"
  Bus Selector2/5 -> Subsystem14/1(<LANE_3_TARGETOBJECT_0_ST>)  "<LANE_3_SEGMENT_4_ST_adp>"
  Bus Selector3/5 -> Bus Creator/6  "<rear_lane_length_f>"
  Bus Selector1/5 -> Subsystem4/1(<LANE_3_TARGETOBJECT_0_ST>)  "<LANE_3_TARGETOBJECT_4_ST>"
  Bus Selector2/6 -> Subsystem15/1(<LANE_3_TARGETOBJECT_0_ST>)  "<LANE_3_SEGMENT_5_ST_adp>"
  Bus Selector1/3 -> Subsystem2/1(<LANE_3_TARGETOBJECT_0_ST>)  "<LANE_3_TARGETOBJECT_2_ST>"
  Bus Selector1/7 -> Subsystem6/1(<LANE_3_TARGETOBJECT_0_ST>)  "<LANE_3_TARGETOBJECT_6_ST>"
  Bus Selector1/9 -> Subsystem8/1(<LANE_3_TARGETOBJECT_0_ST>)  "<LANE_3_TARGETOBJECT_8_ST>"
  Bus Selector/1 -> Bus Selector3/1  "<lane_3>"
  Bus Selector3/2 -> Bus Creator/3  "<available_b>"
  Bus Selector2/3 -> Subsystem12/1(<LANE_3_TARGETOBJECT_0_ST>)  "<LANE_3_SEGMENT_2_ST_adp>"
  Bus Selector1/2 -> Subsystem1/1(<LANE_3_TARGETOBJECT_0_ST>)  "<LANE_3_TARGETOBJECT_1_ST>"
  Subsystem1/1(TARGRTOBJECTS_ST) -> Vector Concatenate/2
  Bus Selector1/10 -> Subsystem9/1(<LANE_3_TARGETOBJECT_0_ST>)  "<LANE_3_TARGETOBJECT_9_ST>"
  Bus Creator/1 -> Out1/1
  Subsystem4/1(TARGRTOBJECTS_ST) -> Vector Concatenate/5
  Subsystem14/1(SEGMENT_ST) -> Vector Concatenate1/5
  Subsystem13/1(SEGMENT_ST) -> Vector Concatenate1/4
  Subsystem5/1(TARGRTOBJECTS_ST) -> Vector Concatenate/6
  Subsystem12/1(SEGMENT_ST) -> Vector Concatenate1/3
  Bus Selector3/3 -> Bus Creator/4  "<lane_dwidth_f>"
  Subsystem6/1(TARGRTOBJECTS_ST) -> Vector Concatenate/7
  Subsystem8/1(TARGRTOBJECTS_ST) -> Vector Concatenate/9
  Subsystem11/1(SEGMENT_ST) -> Vector Concatenate1/2
  Subsystem10/1(SEGMENT_ST) -> Vector Concatenate1/1
  Subsystem2/1(TARGRTOBJECTS_ST) -> Vector Concatenate/3
  Subsystem15/1(SEGMENT_ST) -> Vector Concatenate1/6
  Bus Selector1/8 -> Subsystem7/1(<LANE_3_TARGETOBJECT_0_ST>)  "<LANE_3_TARGETOBJECT_7_ST>"
  Subsystem7/1(TARGRTOBJECTS_ST) -> Vector Concatenate/8
  Subsystem9/1(TARGRTOBJECTS_ST) -> Vector Concatenate/10
  Bus Selector2/4 -> Subsystem13/1(<LANE_3_TARGETOBJECT_0_ST>)  "<LANE_3_SEGMENT_3_ST_adp>"

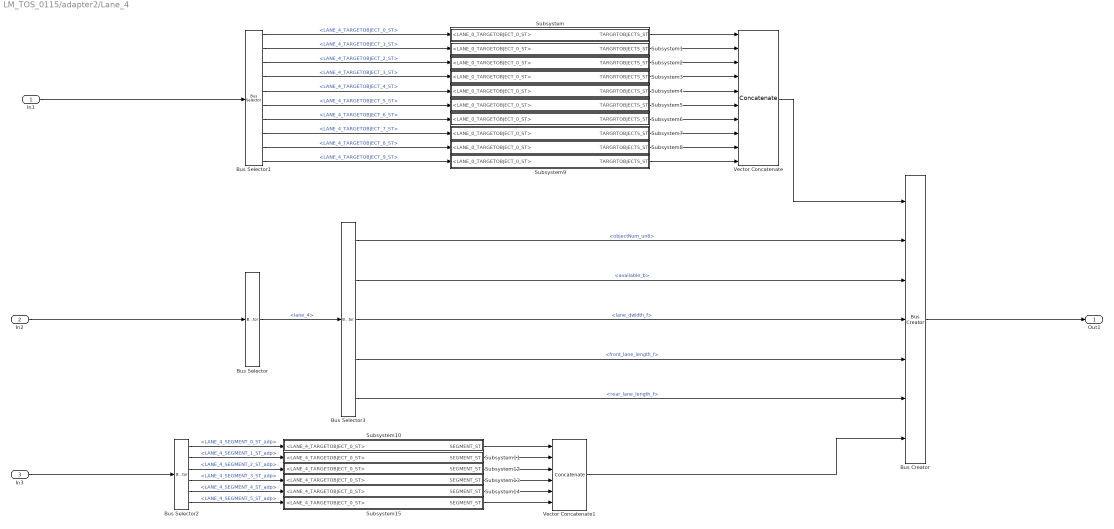
== system LM_TOS_0115/adapter2/Lane_4 ==
  In1 : Inport
  In2 : Inport  Port=2
  In3 : Inport  Port=3
  Bus Creator : BusCreator  Inputs=7  OutDataTypeStr=Bus: LM_LANE_ST  NonVirtualBus=on
  Bus Selector : BusSelector  OutputSignals=lane_4
  Bus Selector1 : BusSelector  OutputSignals=LANE_4_TARGETOBJECT_0_ST,LANE_4_TARGETOBJECT_1_ST,LANE_4_TARGETOBJECT_2_ST,LANE_4_TARGETOBJECT_3_ST,LANE_4_TARGETOBJECT_4_ST,LANE_4_TARGETOBJECT_5_ST,LANE_4_TARGETOBJECT_6_ST,LANE_4_TARGETOBJECT_7_ST,LANE_4_TARGETOBJECT_8_ST,LANE_4_TARGETOBJECT_9_ST
  Bus Selector2 : BusSelector  OutputSignals=LANE_4_SEGMENT_0_ST_adp,LANE_4_SEGMENT_1_ST_adp,LANE_4_SEGMENT_2_ST_adp,LANE_4_SEGMENT_3_ST_adp,LANE_4_SEGMENT_4_ST_adp,LANE_4_SEGMENT_5_ST_adp
  Bus Selector3 : BusSelector  OutputSignals=objectNum_un8,available_b,lane_dwidth_f,front_lane_length_f,rear_lane_length_f
  Subsystem : Subsystem
  Subsystem1 : Subsystem
  Subsystem10 : Subsystem
  Subsystem11 : Subsystem
  Subsystem12 : Subsystem
  Subsystem13 : Subsystem
  Subsystem14 : Subsystem
  Subsystem15 : Subsystem
  Subsystem2 : Subsystem
  Subsystem3 : Subsystem
  Subsystem4 : Subsystem
  Subsystem5 : Subsystem
  Subsystem6 : Subsystem
  Subsystem7 : Subsystem
  Subsystem8 : Subsystem
  Subsystem9 : Subsystem
  Vector Concatenate : Concatenate  NumInputs=10
  Vector Concatenate1 : Concatenate  NumInputs=6
  Out1 : Outport  OutDataTypeStr=Bus: LM_LANE_ST
  wires:
  Bus Selector2/4 -> Subsystem13/1(<LANE_4_TARGETOBJECT_0_ST>)  "<LANE_4_SEGMENT_3_ST_adp>"
  Subsystem9/1(TARGRTOBJECTS_ST) -> Vector Concatenate/10
  Subsystem7/1(TARGRTOBJECTS_ST) -> Vector Concatenate/8
  Bus Selector1/8 -> Subsystem7/1(<LANE_0_TARGETOBJECT_0_ST>)  "<LANE_4_TARGETOBJECT_7_ST>"
  Subsystem15/1(SEGMENT_ST) -> Vector Concatenate1/6
  Subsystem2/1(TARGRTOBJECTS_ST) -> Vector Concatenate/3
  Subsystem10/1(SEGMENT_ST) -> Vector Concatenate1/1
  Subsystem11/1(SEGMENT_ST) -> Vector Concatenate1/2
  Subsystem8/1(TARGRTOBJECTS_ST) -> Vector Concatenate/9
  Subsystem6/1(TARGRTOBJECTS_ST) -> Vector Concatenate/7
  Bus Selector3/3 -> Bus Creator/4  "<lane_dwidth_f>"
  Subsystem12/1(SEGMENT_ST) -> Vector Concatenate1/3
  Subsystem5/1(TARGRTOBJECTS_ST) -> Vector Concatenate/6
  Subsystem13/1(SEGMENT_ST) -> Vector Concatenate1/4
  Subsystem14/1(SEGMENT_ST) -> Vector Concatenate1/5
  Subsystem4/1(TARGRTOBJECTS_ST) -> Vector Concatenate/5
  Bus Creator/1 -> Out1/1
  Bus Selector1/10 -> Subsystem9/1(<LANE_0_TARGETOBJECT_0_ST>)  "<LANE_4_TARGETOBJECT_9_ST>"
  Subsystem1/1(TARGRTOBJECTS_ST) -> Vector Concatenate/2
  Bus Selector1/2 -> Subsystem1/1(<LANE_0_TARGETOBJECT_0_ST>)  "<LANE_4_TARGETOBJECT_1_ST>"
  Bus Selector2/3 -> Subsystem12/1(<LANE_4_TARGETOBJECT_0_ST>)  "<LANE_4_SEGMENT_2_ST_adp>"
  Bus Selector3/2 -> Bus Creator/3  "<available_b>"
  Bus Selector/1 -> Bus Selector3/1  "<lane_4>"
  Bus Selector1/9 -> Subsystem8/1(<LANE_0_TARGETOBJECT_0_ST>)  "<LANE_4_TARGETOBJECT_8_ST>"
  Bus Selector1/7 -> Subsystem6/1(<LANE_0_TARGETOBJECT_0_ST>)  "<LANE_4_TARGETOBJECT_6_ST>"
  Bus Selector1/3 -> Subsystem2/1(<LANE_0_TARGETOBJECT_0_ST>)  "<LANE_4_TARGETOBJECT_2_ST>"
  Bus Selector2/6 -> Subsystem15/1(<LANE_4_TARGETOBJECT_0_ST>)  "<LANE_4_SEGMENT_5_ST_adp>"
  Bus Selector1/5 -> Subsystem4/1(<LANE_0_TARGETOBJECT_0_ST>)  "<LANE_4_TARGETOBJECT_4_ST>"
  Bus Selector3/5 -> Bus Creator/6  "<rear_lane_length_f>"
  Bus Selector2/5 -> Subsystem14/1(<LANE_4_TARGETOBJECT_0_ST>)  "<LANE_4_SEGMENT_4_ST_adp>"
  Bus Selector2/2 -> Subsystem11/1(<LANE_4_TARGETOBJECT_0_ST>)  "<LANE_4_SEGMENT_1_ST_adp>"
  Bus Selector2/1 -> Subsystem10/1(<LANE_4_TARGETOBJECT_0_ST>)  "<LANE_4_SEGMENT_0_ST_adp>"
  In1/1 -> Bus Selector1/1
  In3/1 -> Bus Selector2/1
  Bus Selector1/6 -> Subsystem5/1(<LANE_0_TARGETOBJECT_0_ST>)  "<LANE_4_TARGETOBJECT_5_ST>"
  Bus Selector1/1 -> Subsystem/1(<LANE_0_TARGETOBJECT_0_ST>)  "<LANE_4_TARGETOBJECT_0_ST>"
  Bus Selector1/4 -> Subsystem3/1(<LANE_0_TARGETOBJECT_0_ST>)  "<LANE_4_TARGETOBJECT_3_ST>"
  Bus Selector3/1 -> Bus Creator/2  "<objectNum_un8>"
  Bus Selector3/4 -> Bus Creator/5  "<front_lane_length_f>"
  Subsystem/1(TARGRTOBJECTS_ST) -> Vector Concatenate/1
  Vector Concatenate/1 -> Bus Creator/1
  Subsystem3/1(TARGRTOBJECTS_ST) -> Vector Concatenate/4
  Vector Concatenate1/1 -> Bus Creator/7
  In2/1 -> Bus Selector/1

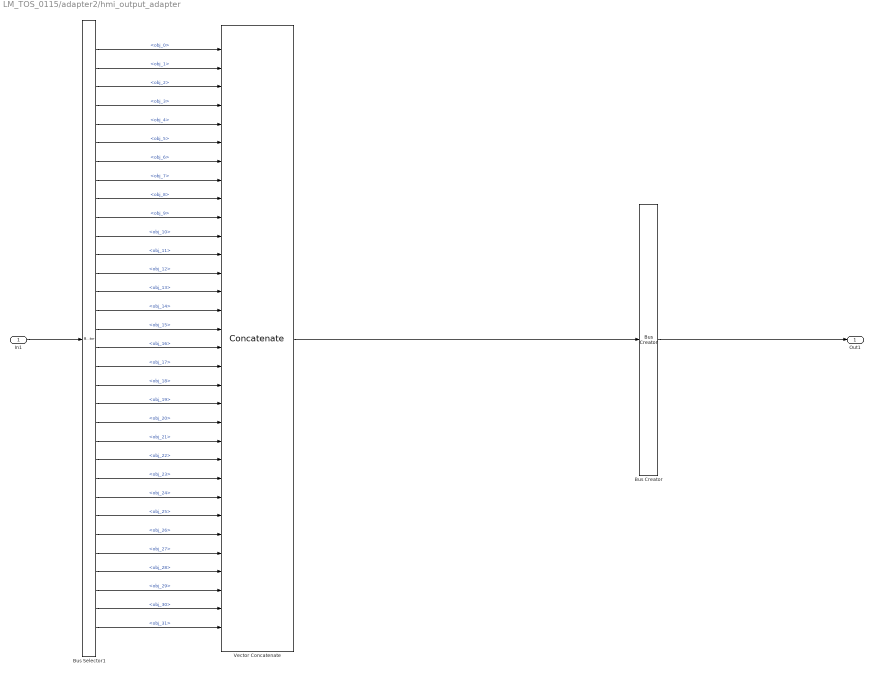
== system LM_TOS_0115/adapter2/hmi_output_adapter ==
  In1 : Inport  OutDataTypeStr=Bus: HMI_OUTPUT_ST_APT
  Bus Creator : BusCreator  Inputs=1  OutDataTypeStr=Bus: HMI_DISPLAY_ARRAY_ST  NonVirtualBus=on
  Bus Selector1 : BusSelector  OutputSignals=obj_0,obj_1,obj_2,obj_3,obj_4,obj_5,obj_6,obj_7,obj_8,obj_9,obj_10,obj_11,obj_12,obj_13,obj_14,obj_15,obj_16,obj_17,obj_18,obj_19,obj_20,obj_21,obj_22,obj_23,obj_24,obj_25,obj_26,obj_27,obj_28,obj_29,obj_30,obj_31
  Vector Concatenate : Concatenate  NumInputs=32
  Out1 : Outport  OutDataTypeStr=Bus: HMI_DISPLAY_ARRAY_ST
  wires:
  Vector Concatenate/1 -> Bus Creator/1
  In1/1 -> Bus Selector1/1
  Bus Creator/1 -> Out1/1
  Bus Selector1/9 -> Vector Concatenate/9  "<obj_8>"
  Bus Selector1/1 -> Vector Concatenate/1  "<obj_0>"
  Bus Selector1/2 -> Vector Concatenate/2  "<obj_1>"
  Bus Selector1/3 -> Vector Concatenate/3  "<obj_2>"
  Bus Selector1/4 -> Vector Concatenate/4  "<obj_3>"
  Bus Selector1/5 -> Vector Concatenate/5  "<obj_4>"
  Bus Selector1/6 -> Vector Concatenate/6  "<obj_5>"
  Bus Selector1/7 -> Vector Concatenate/7  "<obj_6>"
  Bus Selector1/8 -> Vector Concatenate/8  "<obj_7>"
  Bus Selector1/10 -> Vector Concatenate/10  "<obj_9>"
  Bus Selector1/11 -> Vector Concatenate/11  "<obj_10>"
  Bus Selector1/12 -> Vector Concatenate/12  "<obj_11>"
  Bus Selector1/13 -> Vector Concatenate/13  "<obj_12>"
  Bus Selector1/14 -> Vector Concatenate/14  "<obj_13>"
  Bus Selector1/15 -> Vector Concatenate/15  "<obj_14>"
  Bus Selector1/16 -> Vector Concatenate/16  "<obj_15>"
  Bus Selector1/17 -> Vector Concatenate/17  "<obj_16>"
  Bus Selector1/18 -> Vector Concatenate/18  "<obj_17>"
  Bus Selector1/19 -> Vector Concatenate/19  "<obj_18>"
  Bus Selector1/20 -> Vector Concatenate/20  "<obj_19>"
  Bus Selector1/21 -> Vector Concatenate/21  "<obj_20>"
  Bus Selector1/22 -> Vector Concatenate/22  "<obj_21>"
  Bus Selector1/23 -> Vector Concatenate/23  "<obj_22>"
  Bus Selector1/24 -> Vector Concatenate/24  "<obj_23>"
  Bus Selector1/25 -> Vector Concatenate/25  "<obj_24>"
  Bus Selector1/26 -> Vector Concatenate/26  "<obj_25>"
  Bus Selector1/27 -> Vector Concatenate/27  "<obj_26>"
  Bus Selector1/28 -> Vector Concatenate/28  "<obj_27>"
  Bus Selector1/29 -> Vector Concatenate/29  "<obj_28>"
  Bus Selector1/30 -> Vector Concatenate/30  "<obj_29>"
  Bus Selector1/31 -> Vector Concatenate/31  "<obj_30>"
  Bus Selector1/32 -> Vector Concatenate/32  "<obj_31>"

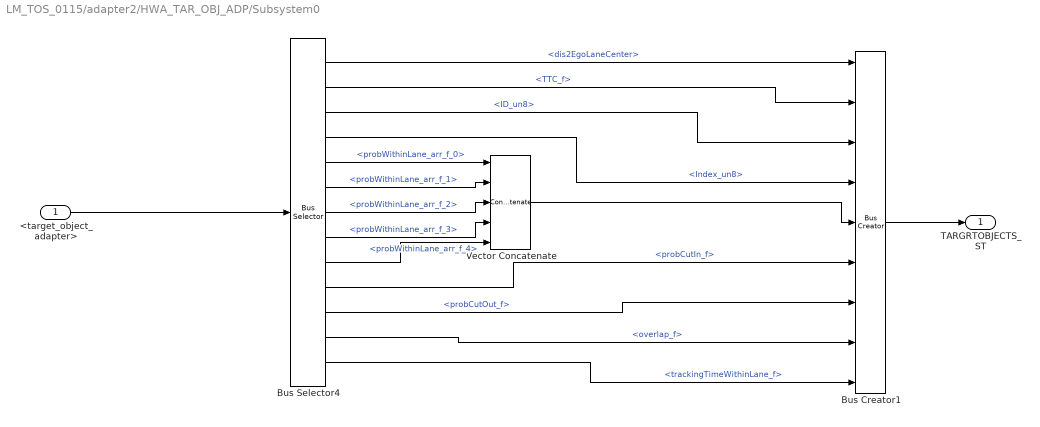
== system LM_TOS_0115/adapter2/HWA_TAR_OBJ_ADP/Subsystem0 ==
  <target_object_adapter> : Inport
  Bus Creator1 : BusCreator  Inputs=9  OutDataTypeStr=Bus: TARGETOBJECT  NonVirtualBus=on
  Bus Selector4 : BusSelector  OutputSignals=dis2EgoLaneCenter,TTC_f,ID_un8,Index_un8,probWithinLane_arr_f_0,probWithinLane_arr_f_1,probWithinLane_arr_f_2,probWithinLane_arr_f_3,probWithinLane_arr_f_4,probCutIn_f,probCutOut_f,overlap_f,trackingTimeWithinLane_f
  Vector Concatenate : Concatenate  NumInputs=5
  TARGRTOBJECTS_ST : Outport  OutDataTypeStr=Bus: TARGETOBJECT
  wires:
  Bus Selector4/8 -> Vector Concatenate/4  "<probWithinLane_arr_f_3>"
  Bus Selector4/11 -> Bus Creator1/7  "<probCutOut_f>"
  Bus Selector4/10 -> Bus Creator1/6  "<probCutIn_f>"
  Bus Selector4/12 -> Bus Creator1/8  "<overlap_f>"
  Bus Selector4/9 -> Vector Concatenate/5  "<probWithinLane_arr_f_4>"
  Bus Selector4/2 -> Bus Creator1/2  "<TTC_f>"
  Bus Selector4/5 -> Vector Concatenate/1  "<probWithinLane_arr_f_0>"
  <target_object_adapter>/1 -> Bus Selector4/1
  Bus Selector4/6 -> Vector Concatenate/2  "<probWithinLane_arr_f_1>"
  Bus Selector4/13 -> Bus Creator1/9  "<trackingTimeWithinLane_f>"
  Bus Selector4/1 -> Bus Creator1/1  "<dis2EgoLaneCenter>"
  Bus Selector4/7 -> Vector Concatenate/3  "<probWithinLane_arr_f_2>"
  Vector Concatenate/1 -> Bus Creator1/5
  Bus Selector4/3 -> Bus Creator1/3  "<ID_un8>"
  Bus Creator1/1 -> TARGRTOBJECTS_ST/1
  Bus Selector4/4 -> Bus Creator1/4  "<Index_un8>"

== system LM_TOS_0115/adapter2/HWA_TAR_OBJ_ADP/Subsystem1 ==
  <target_object_adapter> : Inport
  Bus Creator1 : BusCreator  Inputs=9  OutDataTypeStr=Bus: TARGETOBJECT  NonVirtualBus=on
  Bus Selector4 : BusSelector  OutputSignals=dis2EgoLaneCenter,TTC_f,ID_un8,Index_un8,probWithinLane_arr_f_0,probWithinLane_arr_f_1,probWithinLane_arr_f_2,probWithinLane_arr_f_3,probWithinLane_arr_f_4,probCutIn_f,probCutOut_f,overlap_f,trackingTimeWithinLane_f
  Vector Concatenate : Concatenate  NumInputs=5
  TARGRTOBJECTS_ST : Outport  OutDataTypeStr=Bus: TARGETOBJECT
  wires:
  Bus Selector4/4 -> Bus Creator1/4  "<Index_un8>"
  Bus Creator1/1 -> TARGRTOBJECTS_ST/1
  Bus Selector4/3 -> Bus Creator1/3  "<ID_un8>"
  Vector Concatenate/1 -> Bus Creator1/5
  Bus Selector4/7 -> Vector Concatenate/3  "<probWithinLane_arr_f_2>"
  Bus Selector4/1 -> Bus Creator1/1  "<dis2EgoLaneCenter>"
  Bus Selector4/13 -> Bus Creator1/9  "<trackingTimeWithinLane_f>"
  Bus Selector4/6 -> Vector Concatenate/2  "<probWithinLane_arr_f_1>"
  <target_object_adapter>/1 -> Bus Selector4/1
  Bus Selector4/5 -> Vector Concatenate/1  "<probWithinLane_arr_f_0>"
  Bus Selector4/2 -> Bus Creator1/2  "<TTC_f>"
  Bus Selector4/9 -> Vector Concatenate/5  "<probWithinLane_arr_f_4>"
  Bus Selector4/12 -> Bus Creator1/8  "<overlap_f>"
  Bus Selector4/10 -> Bus Creator1/6  "<probCutIn_f>"
  Bus Selector4/11 -> Bus Creator1/7  "<probCutOut_f>"
  Bus Selector4/8 -> Vector Concatenate/4  "<probWithinLane_arr_f_3>"

== system LM_TOS_0115/adapter2/HWA_TAR_OBJ_ADP/Subsystem10 ==
  <target_object_adapter> : Inport
  Bus Creator1 : BusCreator  Inputs=9  OutDataTypeStr=Bus: TARGETOBJECT  NonVirtualBus=on
  Bus Selector4 : BusSelector  OutputSignals=dis2EgoLaneCenter,TTC_f,ID_un8,Index_un8,probWithinLane_arr_f_0,probWithinLane_arr_f_1,probWithinLane_arr_f_2,probWithinLane_arr_f_3,probWithinLane_arr_f_4,probCutIn_f,probCutOut_f,overlap_f,trackingTimeWithinLane_f
  Vector Concatenate : Concatenate  NumInputs=5
  TARGRTOBJECTS_ST : Outport  OutDataTypeStr=Bus: TARGETOBJECT
  wires:
  Bus Selector4/8 -> Vector Concatenate/4  "<probWithinLane_arr_f_3>"
  Bus Selector4/11 -> Bus Creator1/7  "<probCutOut_f>"
  Bus Selector4/10 -> Bus Creator1/6  "<probCutIn_f>"
  Bus Selector4/12 -> Bus Creator1/8  "<overlap_f>"
  Bus Selector4/9 -> Vector Concatenate/5  "<probWithinLane_arr_f_4>"
  Bus Selector4/2 -> Bus Creator1/2  "<TTC_f>"
  Bus Selector4/5 -> Vector Concatenate/1  "<probWithinLane_arr_f_0>"
  <target_object_adapter>/1 -> Bus Selector4/1
  Bus Selector4/6 -> Vector Concatenate/2  "<probWithinLane_arr_f_1>"
  Bus Selector4/13 -> Bus Creator1/9  "<trackingTimeWithinLane_f>"
  Bus Selector4/1 -> Bus Creator1/1  "<dis2EgoLaneCenter>"
  Bus Selector4/7 -> Vector Concatenate/3  "<probWithinLane_arr_f_2>"
  Vector Concatenate/1 -> Bus Creator1/5
  Bus Selector4/3 -> Bus Creator1/3  "<ID_un8>"
  Bus Creator1/1 -> TARGRTOBJECTS_ST/1
  Bus Selector4/4 -> Bus Creator1/4  "<Index_un8>"

== system LM_TOS_0115/adapter2/HWA_TAR_OBJ_ADP/Subsystem11 ==
  <target_object_adapter> : Inport
  Bus Creator1 : BusCreator  Inputs=9  OutDataTypeStr=Bus: TARGETOBJECT  NonVirtualBus=on
  Bus Selector4 : BusSelector  OutputSignals=dis2EgoLaneCenter,TTC_f,ID_un8,Index_un8,probWithinLane_arr_f_0,probWithinLane_arr_f_1,probWithinLane_arr_f_2,probWithinLane_arr_f_3,probWithinLane_arr_f_4,probCutIn_f,probCutOut_f,overlap_f,trackingTimeWithinLane_f
  Vector Concatenate : Concatenate  NumInputs=5
  TARGRTOBJECTS_ST : Outport  OutDataTypeStr=Bus: TARGETOBJECT
  wires:
  Bus Selector4/4 -> Bus Creator1/4  "<Index_un8>"
  Bus Creator1/1 -> TARGRTOBJECTS_ST/1
  Bus Selector4/3 -> Bus Creator1/3  "<ID_un8>"
  Vector Concatenate/1 -> Bus Creator1/5
  Bus Selector4/7 -> Vector Concatenate/3  "<probWithinLane_arr_f_2>"
  Bus Selector4/1 -> Bus Creator1/1  "<dis2EgoLaneCenter>"
  Bus Selector4/13 -> Bus Creator1/9  "<trackingTimeWithinLane_f>"
  Bus Selector4/6 -> Vector Concatenate/2  "<probWithinLane_arr_f_1>"
  <target_object_adapter>/1 -> Bus Selector4/1
  Bus Selector4/5 -> Vector Concatenate/1  "<probWithinLane_arr_f_0>"
  Bus Selector4/2 -> Bus Creator1/2  "<TTC_f>"
  Bus Selector4/9 -> Vector Concatenate/5  "<probWithinLane_arr_f_4>"
  Bus Selector4/12 -> Bus Creator1/8  "<overlap_f>"
  Bus Selector4/10 -> Bus Creator1/6  "<probCutIn_f>"
  Bus Selector4/11 -> Bus Creator1/7  "<probCutOut_f>"
  Bus Selector4/8 -> Vector Concatenate/4  "<probWithinLane_arr_f_3>"

== system LM_TOS_0115/adapter2/HWA_TAR_OBJ_ADP/Subsystem2 ==
  <target_object_adapter> : Inport
  Bus Creator1 : BusCreator  Inputs=9  OutDataTypeStr=Bus: TARGETOBJECT  NonVirtualBus=on
  Bus Selector4 : BusSelector  OutputSignals=dis2EgoLaneCenter,TTC_f,ID_un8,Index_un8,probWithinLane_arr_f_0,probWithinLane_arr_f_1,probWithinLane_arr_f_2,probWithinLane_arr_f_3,probWithinLane_arr_f_4,probCutIn_f,probCutOut_f,overlap_f,trackingTimeWithinLane_f
  Vector Concatenate : Concatenate  NumInputs=5
  TARGRTOBJECTS_ST : Outport  OutDataTypeStr=Bus: TARGETOBJECT
  wires:
  Bus Selector4/8 -> Vector Concatenate/4  "<probWithinLane_arr_f_3>"
  Bus Selector4/11 -> Bus Creator1/7  "<probCutOut_f>"
  Bus Selector4/10 -> Bus Creator1/6  "<probCutIn_f>"
  Bus Selector4/12 -> Bus Creator1/8  "<overlap_f>"
  Bus Selector4/9 -> Vector Concatenate/5  "<probWithinLane_arr_f_4>"
  Bus Selector4/2 -> Bus Creator1/2  "<TTC_f>"
  Bus Selector4/5 -> Vector Concatenate/1  "<probWithinLane_arr_f_0>"
  <target_object_adapter>/1 -> Bus Selector4/1
  Bus Selector4/6 -> Vector Concatenate/2  "<probWithinLane_arr_f_1>"
  Bus Selector4/13 -> Bus Creator1/9  "<trackingTimeWithinLane_f>"
  Bus Selector4/1 -> Bus Creator1/1  "<dis2EgoLaneCenter>"
  Bus Selector4/7 -> Vector Concatenate/3  "<probWithinLane_arr_f_2>"
  Vector Concatenate/1 -> Bus Creator1/5
  Bus Selector4/3 -> Bus Creator1/3  "<ID_un8>"
  Bus Creator1/1 -> TARGRTOBJECTS_ST/1
  Bus Selector4/4 -> Bus Creator1/4  "<Index_un8>"

== system LM_TOS_0115/adapter2/HWA_TAR_OBJ_ADP/Subsystem3 ==
  <target_object_adapter> : Inport
  Bus Creator1 : BusCreator  Inputs=9  OutDataTypeStr=Bus: TARGETOBJECT  NonVirtualBus=on
  Bus Selector4 : BusSelector  OutputSignals=dis2EgoLaneCenter,TTC_f,ID_un8,Index_un8,probWithinLane_arr_f_0,probWithinLane_arr_f_1,probWithinLane_arr_f_2,probWithinLane_arr_f_3,probWithinLane_arr_f_4,probCutIn_f,probCutOut_f,overlap_f,trackingTimeWithinLane_f
  Vector Concatenate : Concatenate  NumInputs=5
  TARGRTOBJECTS_ST : Outport  OutDataTypeStr=Bus: TARGETOBJECT
  wires:
  Bus Selector4/4 -> Bus Creator1/4  "<Index_un8>"
  Bus Creator1/1 -> TARGRTOBJECTS_ST/1
  Bus Selector4/3 -> Bus Creator1/3  "<ID_un8>"
  Vector Concatenate/1 -> Bus Creator1/5
  Bus Selector4/7 -> Vector Concatenate/3  "<probWithinLane_arr_f_2>"
  Bus Selector4/1 -> Bus Creator1/1  "<dis2EgoLaneCenter>"
  Bus Selector4/13 -> Bus Creator1/9  "<trackingTimeWithinLane_f>"
  Bus Selector4/6 -> Vector Concatenate/2  "<probWithinLane_arr_f_1>"
  <target_object_adapter>/1 -> Bus Selector4/1
  Bus Selector4/5 -> Vector Concatenate/1  "<probWithinLane_arr_f_0>"
  Bus Selector4/2 -> Bus Creator1/2  "<TTC_f>"
  Bus Selector4/9 -> Vector Concatenate/5  "<probWithinLane_arr_f_4>"
  Bus Selector4/12 -> Bus Creator1/8  "<overlap_f>"
  Bus Selector4/10 -> Bus Creator1/6  "<probCutIn_f>"
  Bus Selector4/11 -> Bus Creator1/7  "<probCutOut_f>"
  Bus Selector4/8 -> Vector Concatenate/4  "<probWithinLane_arr_f_3>"
